simulink model "stateFeedbackRegulatorObservationSim"  (R2020a)
settings: Solver=VariableStepAuto  StartTime=0.0  StopTime=Tf  RelTol=1e-9
values from neighbouring files (symbols this model uses):
  A = [0 1 0; 0 0 1; -2 -3 -5]    [stateFeedbackRegulator.m]    (also in stateFeedbackTracking.m; stateObservation.m; stateTrackingPlace.m)
  B = [0; 0; 1]    [stateFeedbackRegulator.m]    (also in stateFeedbackTracking.m; stateObservation.m; stateTrackingPlace.m)
  C = [1 0 0]    [stateFeedbackRegulator.m]    (also in stateFeedbackTracking.m; stateObservation.m; stateTrackingPlace.m)
  K = place(A,B,p_des)    [stateFeedbackPlace.m]    (also in stateFeedbackRegulator.m = [170.8 79.1 9.4]; stateFeedbackTracking.m = Ke(1:3); stateTrackingPlace.m = Ke(1:3))
  L = [L1; L2; L3]    [stateObservation.m]    (also in stateObservationPlace.m = place(A',C',p_des)')
  x0 = [1; 0; 0]    [stateFeedbackRegulator.m]    (also in stateFeedbackRegulatorObservation.m = [2; 5; -1]; stateFeedbackTracking.m = [0; 0; 0]; stateFeedbackTrackingObservation.m = [0; 0; 0]; stateObservation.m = [1; 1; 1])
settings Model: Creator=gbecerra  LastModifiedBy=gbecerra

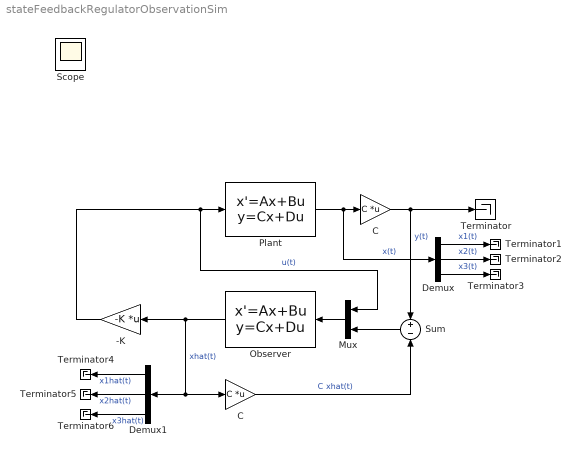
== system stateFeedbackRegulatorObservationSim ==
  -K : Gain  Gain=-K  Multiplication=Matrix(K*u) (u vector)
  C : Gain  Gain=C  Multiplication=Matrix(K*u) (u vector)
  "C " : Gain  Gain=C  Multiplication=Matrix(K*u) (u vector)
  Demux : Demux  Outputs=3
  Demux1 : Demux  Outputs=3
  Mux : Mux  Inputs=2
  Observer : StateSpace  A=A  B=[B L]  C=eye(3)  D=zeros(3,2)  InitialCondition=0
  Plant : StateSpace  A=A  B=B  C=eye(3)  D=zeros(3,1)  InitialCondition=x0
  Sum : Sum  Inputs=+|-
  Terminator{,1..6} (7 alike) : Terminator
  Scope : Scope
  wires:
  Mux/1 -> Observer/1
  -K/1 -> Mux/1, Plant/1  "u(t)"
  Plant/1 -> Demux/1, C/1  "x(t)"
  C/1 -> Terminator/1, Sum/1  "y(t)"
  Observer/1 -> -K/1, Demux1/1, "C "/1  "xhat(t)"
  Sum/1 -> Mux/2
  "C "/1 -> Sum/2  "C xhat(t)"
  Demux/1 -> Terminator1/1  "x1(t)"
  Demux/2 -> Terminator2/1  "x2(t)"
  Demux/3 -> Terminator3/1  "x3(t)"
  Demux1/1 -> Terminator4/1  "x1hat(t)"
  Demux1/2 -> Terminator5/1  "x2hat(t)"
  Demux1/3 -> Terminator6/1  "x3hat(t)"
